simulink model "feedforward1"  (R2015b)
settings: Solver=VariableStepAuto  StartTime=0.0  StopTime=1  RelTol=1e-3
undefined symbols (not defined in the file): den4, num4
libraries: simulink x1
settings Model: Creator=zap  LastModifiedBy=zap

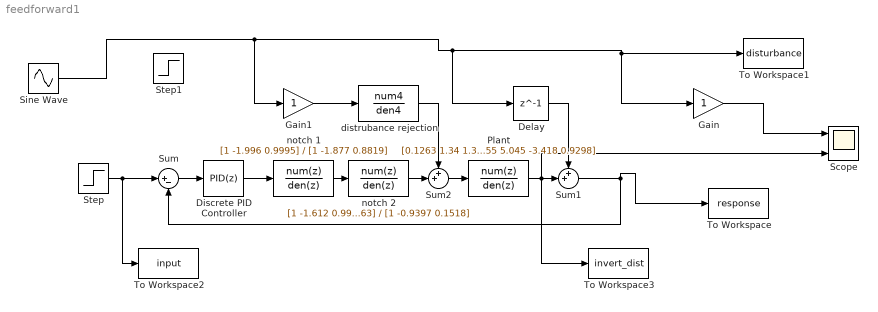
== system feedforward1 ==
  Delay : Delay  DelayLength=1
  Discrete PID Controller : simulink/Continuous/PID Controller  Controller=PID  TimeDomain=Discrete-time  SampleTime=10^-4  IntegratorMethod=Forward Euler  FilterMethod=Forward Euler  Form=Parallel  UseFilter=on  ControllerParametersSource=internal  P=4.1506*10^(-5)  I=0.053132  D=0  N=100  InitialConditionSource=internal  InitialConditionForIntegrator=0  InitialConditionForFilter=0  ExternalReset=none  LimitOutput=off  UpperSaturationLimit=inf  LowerSaturationLimit=-inf  LinearizeAsGain=off  AntiWindupMode=none  Kb=1  TrackingMode=off  Kt=1  PParamMin=[]  PParamMax=[]  IParamMin=[]  IParamMax=[]  DParamMin=[]  DParamMax=[]  NParamMin=[]  NParamMax=[]  KbParamMin=[]  KbParamMax=[]  KtParamMin=[]  KtParamMax=[]  POutMin=[]  POutMax=[]  IOutMin=[]  IOutMax=[]  DOutMin=[]  DOutMax=[]  NOutMin=[]  NOutMax=[]  KbOutMin=[]  KbOutMax=[]  KtOutMin=[]  KtOutMax=[]  IntegratorOutMin=[]  IntegratorOutMax=[]  FilterOutMin=[]  FilterOutMax=[]  SumOutMin=[]  SumOutMax=[]  SumI1OutMin=[]  SumI1OutMax=[]  SumI2OutMin=[]  SumI2OutMax=[]  SumI3OutMin=[]  SumI3OutMax=[]  SumDOutMin=[]  SumDOutMax=[]  SaturationOutMin=[]  SaturationOutMax=[]  IntegratorContinuousStateAttributes=''  IntegratorStateMustResolveToSignalObject=off  IntegratorRTWStateStorageClass=Auto  FilterContinuousStateAttributes=''  FilterStateMustResolveToSignalObject=off  FilterRTWStateStorageClass=Auto  DifferentiatorICPrevScaledInput=0  DifferentiatorOutMin=[]  DifferentiatorOutMax=[]
  Gain : Gain
  Gain1 : Gain
  Plant : DiscreteTransferFcn  Numerator=[0.1263 1.34 1.32 0.1209]  Denominator=[1 -3.555 5.045 -3.418 0.9298]  SampleTime=10^-4
  Scope : Scope  NumInputPorts=3
  Sine Wave : Sin  Amplitude=0.1  Frequency=5000  SampleTime=10^(-4)
  Step : Step  Time=0  SampleTime=10^-4
  Step1 : Step  Time=0  After=0.00001  SampleTime=10^-4
  Sum : Sum  Inputs=|+-
  Sum1 : Sum  Inputs=++|
  Sum2 : Sum  Inputs=++|
  To Workspace : ToWorkspace  VariableName=response  SaveFormat=Timeseries  SampleTime=-1
  To Workspace1 : ToWorkspace  VariableName=disturbance  SaveFormat=Timeseries  SampleTime=-1
  To Workspace2 : ToWorkspace  VariableName=input  SaveFormat=Timeseries  SampleTime=-1
  To Workspace3 : ToWorkspace  VariableName=invert_dist  SaveFormat=Timeseries  SampleTime=-1
  distrubance rejection : DiscreteTransferFcn  Numerator=num4  Denominator=den4  SampleTime=10^-4
  notch 1 : DiscreteTransferFcn  Numerator=[1 -1.996 0.9995]  Denominator=[1 -1.877 0.8819]  SampleTime=10^-4
  notch 2 : DiscreteTransferFcn  Numerator=[1 -1.612 0.9963]  Denominator=[1 -0.9397 0.1518]  SampleTime=10^-4
  wires:
  Sum/1 -> Discrete PID Controller/1
  Discrete PID Controller/1 -> notch 1/1
  notch 1/1 -> notch 2/1
  Step/1 -> To Workspace2/1, Sum/1
  Plant/1 -> To Workspace3/1, Scope/3, Sum1/2
  notch 2/1 -> Sum2/2
  Sum2/1 -> Plant/1
  Gain/1 -> Scope/1
  Delay/1 -> Sum1/1
  Sine Wave/1 -> Gain1/1, Delay/1, To Workspace1/1, Gain/1
  distrubance rejection/1 -> Sum2/1
  Gain1/1 -> distrubance rejection/1
  Sum1/1 -> To Workspace/1, Sum/2
